simulink model "reator_cstr"  (R2021a)
settings: Solver=VariableStepAuto  StartTime=0.0  StopTime=10.0  RelTol=1e-3
settings Model: Creator=Aula  LastModifiedBy=Aula
settings DataIOCC: ReturnWorkspaceOutputs=off

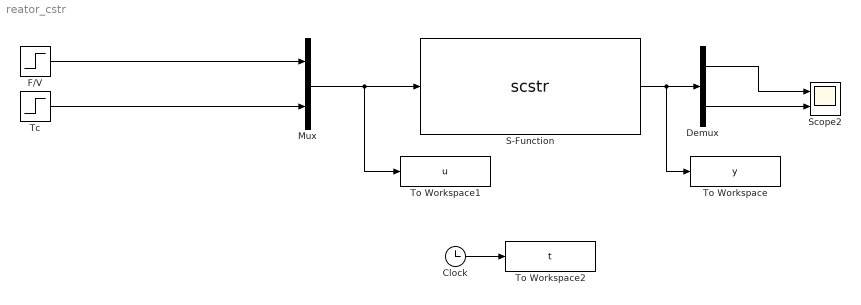
== system reator_cstr ==
  Clock : Clock
  Demux : Demux  Outputs=2
  F/V : Step  Time=0  SampleTime=0
  Mux : Mux  Inputs=2
  S-Function : S-Function  FunctionName=scstr  Parameters=x0model,k0, DeltaE, R, Caf, Tf, ro_Cp, UA_v,neg_DeltaH  SFunctionDeploymentMode=off  EnableBusSupport=off
  Scope2 : Scope  NumInputPorts=2
  Tc : Step  Time=0  After=298  SampleTime=0
  To Workspace : ToWorkspace  VariableName=y  SampleTime=-1
  To Workspace1 : ToWorkspace  VariableName=u  SampleTime=-1
  To Workspace2 : ToWorkspace  VariableName=t  SampleTime=-1
  wires:
  Mux/1 -> To Workspace1/1, S-Function/1
  F/V/1 -> Mux/1
  Tc/1 -> Mux/2
  S-Function/1 -> To Workspace/1, Demux/1
  Demux/1 -> Scope2/1
  Demux/2 -> Scope2/2
  Clock/1 -> To Workspace2/1
